simulink model "ALL_JP360_DBW_V6_5_1103"  (R2022a)
settings: Solver=FixedStepAuto  StartTime=0.0  StopTime=inf  FixedStep=0.01  RelTol=1e-3  EnableMultiTasking=on
model workspace (MAT data in the model file):
  g = 9.8
undefined symbols (not defined in the file or in its folder): canChannel, delta_v_p, IPM_Line_C0, IPM_Line_C1, IPM_Line_C2, IPM_Line_C3, M, M_p, MRR_ObjDistX, MRR_ObjDistY, MRR_ObjFusionCamID, MRR_ObjFusionSig, MRR_ObjID, MRR_ObjRelVelX, MRR_ObjRelVelY, MRR_ObjType, MRR_ObjUpdFlg, none, obj_vaild, untracktime, V, videoinput
libraries: canfdmsglib x230, canfdlib x76, slpidlib x24, simulink x18, dspstat3 x14, ctrlSharedLib x1, simulink_extras x1, imaqlib x1, realtime_pacer_lib x1, dspvision x1, visionsinks x1
(part 27 of 55)

== system ALL_JP360_DBW_V6_5_1103/MsgFromCAN/SRR_ADCU_MsgFromCAN/SRR_ADCU_FRR_OBJPos9_0x1AB ==
  SRR_ADCU_FRR_OBJPos9_0x1ABFromInData : Inport  OutDataTypeStr=Bus:CAN_FD_MESSAGE_BUS
  Bus Creator : BusCreator  Inputs=42  OutDataTypeStr=Bus:SRR_ADCU_FRR_OBJPos9_0x1AB  NonVirtualBus=on
  CAN FD Unpack : canfdmsglib/CAN FD Unpack  CANdbFile=V363 SRR Private CAN-V1.3.dbc  MsgList=(none)  MsgName=FRR_OBJPos9_0x1AB  ProtocolMode=CAN FD  MsgIDType=Standard (11-bit identifier)  MsgIdentifier=427  MsgLength=48  SignalInfo={'FRR_CRCCheck_0x1AB','376','16','BE','unsigned','Standard','0','1','0','0','65535';'FRR_OBJ17_Dx','79','13','BE','unsigned','Standard','0','0.0625','-256','-256','255.938';'FRR_OBJ17_Dy','60','11','BE','unsigned','Standard','0','0.125','-128','-128','127.875';'FRR_OBJ17_ExistProb','112','6','BE','unsigned','Standard','0','2','0','0','100';'FRR_OBJ17_HeadingAngle','55','10','BE','unsigned','Standard','0','0.01','-3.14','-3.14','3.14';'FRR_OBJ17_Height','26','9','BE','unsigned','Standard','0','0.01','0','0','5.11';'FRR_OBJ17_Length','33','9','BE','unsigned','Standard','0','0.05','0','0','25.5';'FRR_OBJ17_Measured','126','2','BE','unsigned','Standard','0','1','0','0','3';'FRR_OBJ17_Motion_Status','162','3','BE','unsigned','Standard','0','1','0','0','7';'FRR_OBJ17_ObstacleProb','120','6','BE','unsigned','Standard','0','2','0','0','100';'FRR_OBJ17_RefPointDx','144','13','BE','unsigned','Standard','0','0.0625','-256','-256','255.938';'FRR_OBJ17_RefPointDy','141','11','BE','unsigned','Standard','0','0.125','-128','-128','127.875';'FRR_OBJ17_RefPointLoc','157','3','BE','unsigned','Standard','0','1','0','0','7';'FRR_OBJ17_RelAx','118','9','BE','unsigned','Standard','0','0.0625','-16','-16','15.9375';'FRR_OBJ17_RelAy','111','10','BE','unsigned','Standard','0','0.03125','-16','-16','15.9688';'FRR_OBJ17_RelVx','89','12','BE','unsigned','Standard','0','0.0625','-128','-128','127.938';'FRR_OBJ17_RelVy','85','10','BE','unsigned','Standard','0','0.125','-64','-64','63.875';'FRR_OBJ17_Track_Age','165','8','BE','unsigned','Standard','0','1','0','0','255';'FRR_OBJ17_Track_ID','1','7','BE','unsigned','Standard','0','1','0','0','127';'FRR_OBJ17_Type','14','3','BE','unsigned','Standard','0','1','0','0','7';'FRR_OBJ17_Width','19','11','BE','unsigned','Standard','0','0.01','0','0','12';'FRR_OBJ18_Dx','247','13','BE','unsigned','Standard','0','0.0625','-256','-256','255.938';'FRR_OBJ18_Dy','228','11','BE','unsigned','Standard','0','0.125','-128','-128','127.875';'FRR_OBJ18_ExistProb','280','6','BE','unsigned','Standard','0','2','0','0','100';'FRR_OBJ18_HeadingAngle','223','10','BE','unsigned','Standard','0','0.01','-3.14','-3.14','3.14';'FRR_OBJ18_Height','194','9','BE','unsigned','Standard','0','0.01','0','0','5.11';'FRR_OBJ18_Length','201','9','BE','unsigned','Standard','0','0.05','0','0','25.5';'FRR_OBJ18_Measured','294','2','BE','unsigned','Standard','0','1','0','0','3';'FRR_OBJ18_Motion_Status','330','3','BE','unsigned','Standard','0','1','0','0','7';'FRR_OBJ18_ObstacleProb','288','6','BE','unsigned','Standard','0','2','0','0','100';'FRR_OBJ18_RefPointDx','312','13','BE','unsigned','Standard','0','0.0625','-256','-256','255.938';'FRR_OBJ18_RefPointDy','309','11','BE','unsigned','Standard','0','0.125','-128','-128','127.875';'FRR_OBJ18_RefPointLoc','325','3','BE','unsigned','Standard','0','1','0','0','7';'FRR_OBJ18_RelAx','286','9','BE','unsigned','Standard','0','0.0625','-16','-16','15.9375';'FRR_OBJ18_RelAy','279','10','BE','unsigned','Standard','0','0.03125','-16','-16','15.9688';'FRR_OBJ18_RelVx','257','12','BE','unsigned','Standard','0','0.0625','-128','-128','127.938';'FRR_OBJ18_RelVy','253','10','BE','unsigned','Standard','0','0.125','-64','-64','63.875';'FRR_OBJ18_Track_Age','333','8','BE','unsigned','Standard','0','1','0','0','255';'FRR_OBJ18_Track_ID','169','7','BE','unsigned','Standard','0','1','0','0','127';'FRR_OBJ18_Type','182','3','BE','unsigned','Standard','0','1','0','0','7';'FRR_OBJ18_Width','187','11','BE','unsigned','Standard','0','0.01','0','0','12';'FRR_RollingCounter_0x1AB','360','4','BE','unsigned','Standard','0','1','0','0','15'}  IDPort=off  TimestampPort=off  ErrorPort=off  RemotePort=off  LengthPort=off  StatusPort=off  BRSPort=off  ESIPort=off  DLCPort=off  ApplyMinMax=off
      settings: SourceProductBaseCode=ME,XP,VN  DataFormat=CANdb specified signals
  Data Type Conversion1 : DataTypeConversion  OutDataTypeStr=uint16  SaturateOnIntegerOverflow=off  RndMeth=Floor
  Data Type Conversion{4,8..10,13,19..20,24,28..30,33,39..40,42} (15 alike) : DataTypeConversion  OutDataTypeStr=int8  SaturateOnIntegerOverflow=off  RndMeth=Floor
  Data Type Conversion{2..3,5..7,11..12,14..17,21..23,25..27,31..32,34..37,41} (24 alike) : DataTypeConversion  OutDataTypeStr=single  SaturateOnIntegerOverflow=off  RndMeth=Floor
  Data Type Conversion18 : DataTypeConversion  OutDataTypeStr=uint8  SaturateOnIntegerOverflow=off  RndMeth=Floor
  Data Type Conversion38 : DataTypeConversion  OutDataTypeStr=uint8  SaturateOnIntegerOverflow=off  RndMeth=Floor
  SRR_ADCU_FRR_OBJPos9_0x1ABFromOutData : Outport  OutDataTypeStr=Bus:SRR_ADCU_FRR_OBJPos9_0x1AB
  wires:
  CAN FD Unpack/1 -> Data Type Conversion1/1
  CAN FD Unpack/2 -> Data Type Conversion2/1
  CAN FD Unpack/3 -> Data Type Conversion3/1
  CAN FD Unpack/4 -> Data Type Conversion4/1
  CAN FD Unpack/5 -> Data Type Conversion5/1
  CAN FD Unpack/6 -> Data Type Conversion6/1
  CAN FD Unpack/7 -> Data Type Conversion7/1
  CAN FD Unpack/8 -> Data Type Conversion8/1
  CAN FD Unpack/9 -> Data Type Conversion9/1
  CAN FD Unpack/10 -> Data Type Conversion10/1
  CAN FD Unpack/11 -> Data Type Conversion11/1
  CAN FD Unpack/12 -> Data Type Conversion12/1
  CAN FD Unpack/13 -> Data Type Conversion13/1
  CAN FD Unpack/14 -> Data Type Conversion14/1
  CAN FD Unpack/15 -> Data Type Conversion15/1
  CAN FD Unpack/16 -> Data Type Conversion16/1
  CAN FD Unpack/17 -> Data Type Conversion17/1
  CAN FD Unpack/18 -> Data Type Conversion18/1
  CAN FD Unpack/19 -> Data Type Conversion19/1
  CAN FD Unpack/20 -> Data Type Conversion20/1
  CAN FD Unpack/21 -> Data Type Conversion21/1
  CAN FD Unpack/22 -> Data Type Conversion22/1
  CAN FD Unpack/23 -> Data Type Conversion23/1
  CAN FD Unpack/24 -> Data Type Conversion24/1
  CAN FD Unpack/25 -> Data Type Conversion25/1
  CAN FD Unpack/26 -> Data Type Conversion26/1
  CAN FD Unpack/27 -> Data Type Conversion27/1
  CAN FD Unpack/28 -> Data Type Conversion28/1
  CAN FD Unpack/29 -> Data Type Conversion29/1
  CAN FD Unpack/30 -> Data Type Conversion30/1
  CAN FD Unpack/31 -> Data Type Conversion31/1
  CAN FD Unpack/32 -> Data Type Conversion32/1
  CAN FD Unpack/33 -> Data Type Conversion33/1
  CAN FD Unpack/34 -> Data Type Conversion34/1
  CAN FD Unpack/35 -> Data Type Conversion35/1
  CAN FD Unpack/36 -> Data Type Conversion36/1
  CAN FD Unpack/37 -> Data Type Conversion37/1
  CAN FD Unpack/38 -> Data Type Conversion38/1
  CAN FD Unpack/39 -> Data Type Conversion39/1
  CAN FD Unpack/40 -> Data Type Conversion40/1
  CAN FD Unpack/41 -> Data Type Conversion41/1
  CAN FD Unpack/42 -> Data Type Conversion42/1
  Data Type Conversion1/1 -> Bus Creator/1  "FRR_CRCCheck_0x1AB"
  Data Type Conversion2/1 -> Bus Creator/2  "FRR_OBJ17_Dx"
  Data Type Conversion3/1 -> Bus Creator/3  "FRR_OBJ17_Dy"
  Data Type Conversion4/1 -> Bus Creator/4  "FRR_OBJ17_ExistProb"
  Data Type Conversion5/1 -> Bus Creator/5  "FRR_OBJ17_HeadingAngle"
  Data Type Conversion6/1 -> Bus Creator/6  "FRR_OBJ17_Height"
  Data Type Conversion7/1 -> Bus Creator/7  "FRR_OBJ17_Length"
  Data Type Conversion8/1 -> Bus Creator/8  "FRR_OBJ17_Measured"
  Data Type Conversion9/1 -> Bus Creator/9  "FRR_OBJ17_Motion_Status"
  Data Type Conversion10/1 -> Bus Creator/10  "FRR_OBJ17_ObstacleProb"
  Data Type Conversion11/1 -> Bus Creator/11  "FRR_OBJ17_RefPointDx"
  Data Type Conversion12/1 -> Bus Creator/12  "FRR_OBJ17_RefPointDy"
  Data Type Conversion13/1 -> Bus Creator/13  "FRR_OBJ17_RefPointLoc"
  Data Type Conversion14/1 -> Bus Creator/14  "FRR_OBJ17_RelAx"
  Data Type Conversion15/1 -> Bus Creator/15  "FRR_OBJ17_RelAy"
  Data Type Conversion16/1 -> Bus Creator/16  "FRR_OBJ17_RelVx"
  Data Type Conversion17/1 -> Bus Creator/17  "FRR_OBJ17_RelVy"
  Data Type Conversion18/1 -> Bus Creator/18  "FRR_OBJ17_Track_Age"
  Data Type Conversion19/1 -> Bus Creator/19  "FRR_OBJ17_Track_ID"
  Data Type Conversion20/1 -> Bus Creator/20  "FRR_OBJ17_Type"
  Data Type Conversion21/1 -> Bus Creator/21  "FRR_OBJ17_Width"
  Data Type Conversion22/1 -> Bus Creator/22  "FRR_OBJ18_Dx"
  Data Type Conversion23/1 -> Bus Creator/23  "FRR_OBJ18_Dy"
  Data Type Conversion24/1 -> Bus Creator/24  "FRR_OBJ18_ExistProb"
  Data Type Conversion25/1 -> Bus Creator/25  "FRR_OBJ18_HeadingAngle"
  Data Type Conversion26/1 -> Bus Creator/26  "FRR_OBJ18_Height"
  Data Type Conversion27/1 -> Bus Creator/27  "FRR_OBJ18_Length"
  Data Type Conversion28/1 -> Bus Creator/28  "FRR_OBJ18_Measured"
  Data Type Conversion29/1 -> Bus Creator/29  "FRR_OBJ18_Motion_Status"
  Data Type Conversion30/1 -> Bus Creator/30  "FRR_OBJ18_ObstacleProb"
  Data Type Conversion31/1 -> Bus Creator/31  "FRR_OBJ18_RefPointDx"
  Data Type Conversion32/1 -> Bus Creator/32  "FRR_OBJ18_RefPointDy"
  Data Type Conversion33/1 -> Bus Creator/33  "FRR_OBJ18_RefPointLoc"
  Data Type Conversion34/1 -> Bus Creator/34  "FRR_OBJ18_RelAx"
  Data Type Conversion35/1 -> Bus Creator/35  "FRR_OBJ18_RelAy"
  Data Type Conversion36/1 -> Bus Creator/36  "FRR_OBJ18_RelVx"
  Data Type Conversion37/1 -> Bus Creator/37  "FRR_OBJ18_RelVy"
  Data Type Conversion38/1 -> Bus Creator/38  "FRR_OBJ18_Track_Age"
  Data Type Conversion39/1 -> Bus Creator/39  "FRR_OBJ18_Track_ID"
  Data Type Conversion40/1 -> Bus Creator/40  "FRR_OBJ18_Type"
  Data Type Conversion41/1 -> Bus Creator/41  "FRR_OBJ18_Width"
  Data Type Conversion42/1 -> Bus Creator/42  "FRR_RollingCounter_0x1AB"
  Bus Creator/1 -> SRR_ADCU_FRR_OBJPos9_0x1ABFromOutData/1  "SRR_ADCU_FRR_OBJPos9_0x1ABFromOutData"
  SRR_ADCU_FRR_OBJPos9_0x1ABFromInData/1 -> CAN FD Unpack/1  "SRR_ADCU_FRR_OBJPos9_0x1ABFromInData"

== system ALL_JP360_DBW_V6_5_1103/MsgFromCAN/SRR_ADCU_MsgFromCAN/SRR_ADCU_RLR_AssistSysSt_0x74 ==
  SRR_ADCU_RLR_AssistSysSt_0x74FromInData : Inport  OutDataTypeStr=Bus:CAN_FD_MESSAGE_BUS
  Bus Creator : BusCreator  Inputs=11  OutDataTypeStr=Bus:SRR_ADCU_RLR_AssistSysSt_0x74  NonVirtualBus=on
  CAN FD Unpack : canfdmsglib/CAN FD Unpack  CANdbFile=V363 SRR Private CAN-V1.3.dbc  MsgList=(none)  MsgName=RLR_AssistSysSt_0x74  ProtocolMode=CAN FD  MsgIDType=Standard (11-bit identifier)  MsgIdentifier=116  MsgLength=20  SignalInfo={'RLR_CRCCheck_RLR_AssistSysSt','152','16','BE','unsigned','Standard','0','1','0','0','65535';'RLR_Localtime_Nsec','122','30','BE','unsigned','Standard','0','1','0','0','1073741823';'RLR_Localtime_sec','48','32','BE','unsigned','Standard','0','1','0','0','4294967295';'RLR_RCTBTargetDecel','76','16','BE','unsigned','Standard','0','0.0005','-16','-16','16';'RLR_RCTB_req','60','1','BE','unsigned','Standard','0','1','0','0','1';'RLR_RollingCounter_RLR_AssistSysSt','136','4','BE','unsigned','Standard','0','1','0','0','15';'RLR_SRR_Obj_Failure','5','3','BE','unsigned','Standard','0','1','0','0','7';'RLR_SRR_TiBas','63','1','BE','unsigned','Standard','0','1','0','0','1';'RLR_SRR_TiLeap','62','1','BE','unsigned','Standard','0','1','0','0','1';'RLR_SRR_TiOut','61','1','BE','unsigned','Standard','0','1','0','0','1';'RLR_SRR_alignAngle','8','13','BE','unsigned','Standard','0','0.01','0','0','80'}  IDPort=off  TimestampPort=off  ErrorPort=off  RemotePort=off  LengthPort=off  StatusPort=off  BRSPort=off  ESIPort=off  DLCPort=off  ApplyMinMax=off
      settings: SourceProductBaseCode=ME,XP,VN  DataFormat=CANdb specified signals
  Data Type Conversion1 : DataTypeConversion  OutDataTypeStr=uint16  SaturateOnIntegerOverflow=off  RndMeth=Floor
  Data Type Conversion{5,8..10} (4 alike) : DataTypeConversion  OutDataTypeStr=boolean  SaturateOnIntegerOverflow=off  RndMeth=Floor
  Data Type Conversion11 : DataTypeConversion  OutDataTypeStr=single  SaturateOnIntegerOverflow=off  RndMeth=Floor
  Data Type Conversion2 : DataTypeConversion  OutDataTypeStr=int32  SaturateOnIntegerOverflow=off  RndMeth=Floor
  Data Type Conversion3 : DataTypeConversion  OutDataTypeStr=uint32  SaturateOnIntegerOverflow=off  RndMeth=Floor
  Data Type Conversion4 : DataTypeConversion  OutDataTypeStr=single  SaturateOnIntegerOverflow=off  RndMeth=Floor
  Data Type Conversion6 : DataTypeConversion  OutDataTypeStr=int8  SaturateOnIntegerOverflow=off  RndMeth=Floor
  Data Type Conversion7 : DataTypeConversion  OutDataTypeStr=int8  SaturateOnIntegerOverflow=off  RndMeth=Floor
  SRR_ADCU_RLR_AssistSysSt_0x74FromOutData : Outport  OutDataTypeStr=Bus:SRR_ADCU_RLR_AssistSysSt_0x74
  wires:
  CAN FD Unpack/1 -> Data Type Conversion1/1
  CAN FD Unpack/2 -> Data Type Conversion2/1
  CAN FD Unpack/3 -> Data Type Conversion3/1
  CAN FD Unpack/4 -> Data Type Conversion4/1
  CAN FD Unpack/5 -> Data Type Conversion5/1
  CAN FD Unpack/6 -> Data Type Conversion6/1
  CAN FD Unpack/7 -> Data Type Conversion7/1
  CAN FD Unpack/8 -> Data Type Conversion8/1
  CAN FD Unpack/9 -> Data Type Conversion9/1
  CAN FD Unpack/10 -> Data Type Conversion10/1
  CAN FD Unpack/11 -> Data Type Conversion11/1
  Data Type Conversion1/1 -> Bus Creator/1  "RLR_CRCCheck_RLR_AssistSysSt"
  Data Type Conversion2/1 -> Bus Creator/2  "RLR_Localtime_Nsec"
  Data Type Conversion3/1 -> Bus Creator/3  "RLR_Localtime_sec"
  Data Type Conversion4/1 -> Bus Creator/4  "RLR_RCTBTargetDecel"
  Data Type Conversion5/1 -> Bus Creator/5  "RLR_RCTB_req"
  Data Type Conversion6/1 -> Bus Creator/6  "RLR_RollingCounter_RLR_AssistSysSt"
  Data Type Conversion7/1 -> Bus Creator/7  "RLR_SRR_Obj_Failure"
  Data Type Conversion8/1 -> Bus Creator/8  "RLR_SRR_TiBas"
  Data Type Conversion9/1 -> Bus Creator/9  "RLR_SRR_TiLeap"
  Data Type Conversion10/1 -> Bus Creator/10  "RLR_SRR_TiOut"
  Data Type Conversion11/1 -> Bus Creator/11  "RLR_SRR_alignAngle"
  Bus Creator/1 -> SRR_ADCU_RLR_AssistSysSt_0x74FromOutData/1  "SRR_ADCU_RLR_AssistSysSt_0x74FromOutData"
  SRR_ADCU_RLR_AssistSysSt_0x74FromInData/1 -> CAN FD Unpack/1  "SRR_ADCU_RLR_AssistSysSt_0x74FromInData"

== system ALL_JP360_DBW_V6_5_1103/MsgFromCAN/SRR_ADCU_MsgFromCAN/SRR_ADCU_RLR_Freespace_0x1F1 ==
  SRR_ADCU_RLR_Freespace_0x1F1FromInData : Inport  OutDataTypeStr=Bus:CAN_FD_MESSAGE_BUS
  Bus Creator : BusCreator  Inputs=104  OutDataTypeStr=Bus:SRR_ADCU_RLR_Freespace_0x1F1  NonVirtualBus=on
  CAN FD Unpack : canfdmsglib/CAN FD Unpack  CANdbFile=V363 SRR Private CAN-V1.3.dbc  MsgList=(none)  MsgName=RLR_Freespace_0x1F1  ProtocolMode=CAN FD  MsgIDType=Standard (11-bit identifier)  MsgIdentifier=497  MsgLength=64  SignalInfo={'RLR_CRCCheck_FSP_MSG1','504','16','BE','unsigned','Standard','0','1','0','0','65535';'RLR_FreespaceSectorConfidence1','12','2','BE','unsigned','Standard','0','1','0','0','3';'RLR_FreespaceSectorConfidence10','142','2','BE','unsigned','Standard','0','1','0','0','3';'RLR_FreespaceSectorConfidence11','144','2','BE','unsigned','Standard','0','1','0','0','3';'RLR_FreespaceSectorConfidence12','162','2','BE','unsigned','Standard','0','1','0','0','3';'RLR_FreespaceSectorConfidence13','180','2','BE','unsigned','Standard','0','1','0','0','3';'RLR_FreespaceSectorConfidence14','198','2','BE','unsigned','Standard','0','1','0','0','3';'RLR_FreespaceSectorConfidence15','200','2','BE','unsigned','Standard','0','1','0','0','3';'RLR_FreespaceSectorConfidence16','218','2','BE','unsigned','Standard','0','1','0','0','3';'RLR_FreespaceSectorConfidence17','236','2','BE','unsigned','Standard','0','1','0','0','3';'RLR_FreespaceSectorConfidence18','254','2','BE','unsigned','Standard','0','1','0','0','3';'RLR_FreespaceSectorConfidence19','256','2','BE','unsigned','Standard','0','1','0','0','3';'RLR_FreespaceSectorConfidence2','30','2','BE','unsigned','Standard','0','1','0','0','3';'RLR_FreespaceSectorConfidence20','274','2','BE','unsigned','Standard','0','1','0','0','3';'RLR_FreespaceSectorConfidence21','292','2','BE','unsigned','Standard','0','1','0','0','3';'RLR_FreespaceSectorConfidence22','310','2','BE','unsigned','Standard','0','1','0','0','3';'RLR_FreespaceSectorConfidence23','312','2','BE','unsigned','Standard','0','1','0','0','3';'RLR_FreespaceSectorConfidence24','330','2','BE','unsigned','Standard','0','1','0','0','3';'RLR_FreespaceSectorConfidence25','348','2','BE','unsigned','Standard','0','1','0','0','3';'RLR_FreespaceSectorConfidence26','366','2','BE','unsigned','Standard','0','1','0','0','3';'RLR_FreespaceSectorConfidence27','368','2','BE','unsigned','Standard','0','1','0','0','3';'RLR_FreespaceSectorConfidence28','386','2','BE','unsigned','Standard','0','1','0','0','3';'RLR_FreespaceSectorConfidence29','404','2','BE','unsigned','Standard','0','1','0','0','3';'RLR_FreespaceSectorConfidence3','32','2','BE','unsigned','Standard','0','1','0','0','3';'RLR_FreespaceSectorConfidence30','422','2','BE','unsigned','Standard','0','1','0','0','3';'RLR_FreespaceSectorConfidence31','424','2','BE','unsigned','Standard','0','1','0','0','3';'RLR_FreespaceSectorConfidence32','442','2','BE','unsigned','Standard','0','1','0','0','3';'RLR_FreespaceSectorConfidence33','460','2','BE','unsigned','Standard','0','1','0','0','3';'RLR_FreespaceSectorConfidence34','478','2','BE','unsigned','Standard','0','1','0','0','3';'RLR_FreespaceSectorConfidence4','50','2','BE','unsigned','Standard','0','1','0','0','3';'RLR_FreespaceSectorConfidence5','68','2','BE','unsigned','Standard','0','1','0','0','3';'RLR_FreespaceSectorConfidence6','86','2','BE','unsigned','Standard','0','1','0','0','3';'RLR_FreespaceSectorConfidence7','88','2','BE','unsigned','Standard','0','1','0','0','3';'RLR_FreespaceSectorConfidence8','106','2','BE','unsigned','Standard','0','1','0','0','3';'RLR_FreespaceSectorConfidence9','124','2','BE','unsigned','Standard','0','1','0','0','3';'RLR_FreespaceSectorDistance1','14','10','BE','unsigned','Standard','0','0.1','0','0','100';'RLR_FreespaceSectorDistance10','128','10','BE','unsigned','Standard','0','0.1','0','0','100';'RLR_FreespaceSectorDistance11','146','10','BE','unsigned','Standard','0','0.1','0','0','100';'RLR_FreespaceSectorDistance12','164','10','BE','unsigned','Standard','0','0.1','0','0','100';'RLR_FreespaceSectorDistance13','182','10','BE','unsigned','Standard','0','0.1','0','0','100';'RLR_FreespaceSectorDistance14','184','10','BE','unsigned','Standard','0','0.1','0','0','100';'RLR_FreespaceSectorDistance15','202','10','BE','unsigned','Standard','0','0.1','0','0','100';'RLR_FreespaceSectorDistance16','220','10','BE','unsigned','Standard','0','0.1','0','0','100';'RLR_FreespaceSectorDistance17','238','10','BE','unsigned','Standard','0','0.1','0','0','100';'RLR_FreespaceSectorDistance18','240','10','BE','unsigned','Standard','0','0.1','0','0','100';'RLR_FreespaceSectorDistance19','258','10','BE','unsigned','Standard','0','0.1','0','0','100';'RLR_FreespaceSectorDistance2','16','10','BE','unsigned','Standard','0','0.1','0','0','100';'RLR_FreespaceSectorDistance20','276','10','BE','unsigned','Standard','0','0.1','0','0','100';'RLR_FreespaceSectorDistance21','294','10','BE','unsigned','Standard','0','0.1','0','0','100';'RLR_FreespaceSectorDistance22','296','10','BE','unsigned','Standard','0','0.1','0','0','100';'RLR_FreespaceSectorDistance23','314','10','BE','unsigned','Standard','0','0.1','0','0','100';'RLR_FreespaceSectorDistance24','332','10','BE','unsigned','Standard','0','0.1','0','0','100';'RLR_FreespaceSectorDistance25','350','10','BE','unsigned','Standard','0','0.1','0','0','100';'RLR_FreespaceSectorDistance26','352','10','BE','unsigned','Standard','0','0.1','0','0','100';'RLR_FreespaceSectorDistance27','370','10','BE','unsigned','Standard','0','0.1','0','0','100';'RLR_FreespaceSectorDistance28','388','10','BE','unsigned','Standard','0','0.1','0','0','100';'RLR_FreespaceSectorDistance29','406','10','BE','unsigned','Standard','0','0.1','0','0','100';'RLR_FreespaceSectorDistance3','34','10','BE','unsigned','Standard','0','0.1','0','0','100';'RLR_FreespaceSectorDistance30','408','10','BE','unsigned','Standard','0','0.1','0','0','100';'RLR_FreespaceSectorDistance31','426','10','BE','unsigned','Standard','0','0.1','0','0','100';'RLR_FreespaceSectorDistance32','444','10','BE','unsigned','Standard','0','0.1','0','0','100';'RLR_FreespaceSectorDistance33','462','10','BE','unsigned','Standard','0','0.1','0','0','100';'RLR_FreespaceSectorDistance34','464','10','BE','unsigned','Standard','0','0.1','0','0','100';'RLR_FreespaceSectorDistance4','52','10','BE','unsigned','Standard','0','0.1','0','0','100';'RLR_FreespaceSectorDistance5','70','10','BE','unsigned','Standard','0','0.1','0','0','100';'RLR_FreespaceSectorDistance6','72','10','BE','unsigned','Standard','0','0.1','0','0','100';'RLR_FreespaceSectorDistance7','90','10','BE','unsigned','Standard','0','0.1','0','0','100';'RLR_FreespaceSectorDistance8','108','10','BE','unsigned','Standard','0','0.1','0','0','100';'RLR_FreespaceSectorDistance9','126','10','BE','unsigned','Standard','0','0.1','0','0','100';'RLR_FreespaceSectorKinestate1','10','2','BE','unsigned','Standard','0','1','0','0','3';'RLR_FreespaceSectorKinestate10','140','2','BE','unsigned','Standard','0','1','0','0','3';'RLR_FreespaceSectorKinestate11','158','2','BE','unsigned','Standard','0','1','0','0','3';'RLR_FreespaceSectorKinestate12','160','2','BE','unsigned','Standard','0','1','0','0','3';'RLR_FreespaceSectorKinestate13','178','2','BE','unsigned','Standard','0','1','0','0','3';'RLR_FreespaceSectorKinestate14','196','2','BE','unsigned','Standard','0','1','0','0','3';'RLR_FreespaceSectorKinestate15','214','2','BE','unsigned','Standard','0','1','0','0','3';'RLR_FreespaceSectorKinestate16','216','2','BE','unsigned','Standard','0','1','0','0','3';'RLR_FreespaceSectorKinestate17','234','2','BE','unsigned','Standard','0','1','0','0','3';'RLR_FreespaceSectorKinestate18','252','2','BE','unsigned','Standard','0','1','0','0','3';'RLR_FreespaceSectorKinestate19','270','2','BE','unsigned','Standard','0','1','0','0','3';'RLR_FreespaceSectorKinestate2','28','2','BE','unsigned','Standard','0','1','0','0','3';'RLR_FreespaceSectorKinestate20','272','2','BE','unsigned','Standard','0','1','0','0','3';'RLR_FreespaceSectorKinestate21','290','2','BE','unsigned','Standard','0','1','0','0','3';'RLR_FreespaceSectorKinestate22','308','2','BE','unsigned','Standard','0','1','0','0','3';'RLR_FreespaceSectorKinestate23','326','2','BE','unsigned','Standard','0','1','0','0','3';'RLR_FreespaceSectorKinestate24','328','2','BE','unsigned','Standard','0','1','0','0','3';'RLR_FreespaceSectorKinestate25','346','2','BE','unsigned','Standard','0','1','0','0','3';'RLR_FreespaceSectorKinestate26','364','2','BE','unsigned','Standard','0','1','0','0','3';'RLR_FreespaceSectorKinestate27','382','2','BE','unsigned','Standard','0','1','0','0','3';'RLR_FreespaceSectorKinestate28','384','2','BE','unsigned','Standard','0','1','0','0','3';'RLR_FreespaceSectorKinestate29','402','2','BE','unsigned','Standard','0','1','0','0','3';'RLR_FreespaceSectorKinestate3','46','2','BE','unsigned','Standard','0','1','0','0','3';'RLR_FreespaceSectorKinestate30','420','2','BE','unsigned','Standard','0','1','0','0','3';'RLR_FreespaceSectorKinestate31','438','2','BE','unsigned','Standard','0','1','0','0','3';'RLR_FreespaceSectorKinestate32','440','2','BE','unsigned','Standard','0','1','0','0','3';'RLR_FreespaceSectorKinestate33','458','2','BE','unsigned','Standard','0','1','0','0','3';'RLR_FreespaceSectorKinestate34','476','2','BE','unsigned','Standard','0','1','0','0','3';'RLR_FreespaceSectorKinestate4','48','2','BE','unsigned','Standard','0','1','0','0','3';'RLR_FreespaceSectorKinestate5','66','2','BE','unsigned','Standard','0','1','0','0','3';'RLR_FreespaceSectorKinestate6','84','2','BE','unsigned','Standard','0','1','0','0','3';'RLR_FreespaceSectorKinestate7','102','2','BE','unsigned','Standard','0','1','0','0','3';'RLR_FreespaceSectorKinestate8','104','2','BE','unsigned','Standard','0','1','0','0','3';'RLR_FreespaceSectorKinestate9','122','2','BE','unsigned','Standard','0','1','0','0','3';'RLR_RollingCounter_FSP_MSG1','488','4','BE','unsigned','Standard','0','1','0','0','15'}  IDPort=off  TimestampPort=off  ErrorPort=off  RemotePort=off  LengthPort=off  StatusPort=off  BRSPort=off  ESIPort=off  DLCPort=off  ApplyMinMax=off
      settings: SourceProductBaseCode=ME,XP,VN  DataFormat=CANdb specified signals
  Data Type Conversion1 : DataTypeConversion  OutDataTypeStr=uint16  SaturateOnIntegerOverflow=off  RndMeth=Floor
  Data Type Conversion{2..35,70..104} (69 alike) : DataTypeConversion  OutDataTypeStr=int8  SaturateOnIntegerOverflow=off  RndMeth=Floor
  Data Type Conversion{36..69} (34 alike) : DataTypeConversion  OutDataTypeStr=single  SaturateOnIntegerOverflow=off  RndMeth=Floor
  SRR_ADCU_RLR_Freespace_0x1F1FromOutData : Outport  OutDataTypeStr=Bus:SRR_ADCU_RLR_Freespace_0x1F1
  wires:
  CAN FD Unpack/1 -> Data Type Conversion1/1
  CAN FD Unpack/2 -> Data Type Conversion2/1
  CAN FD Unpack/3 -> Data Type Conversion3/1
  CAN FD Unpack/4 -> Data Type Conversion4/1
  CAN FD Unpack/5 -> Data Type Conversion5/1
  CAN FD Unpack/6 -> Data Type Conversion6/1
  CAN FD Unpack/7 -> Data Type Conversion7/1
  CAN FD Unpack/8 -> Data Type Conversion8/1
  CAN FD Unpack/9 -> Data Type Conversion9/1
  CAN FD Unpack/10 -> Data Type Conversion10/1
  CAN FD Unpack/11 -> Data Type Conversion11/1
  CAN FD Unpack/12 -> Data Type Conversion12/1
  CAN FD Unpack/13 -> Data Type Conversion13/1
  CAN FD Unpack/14 -> Data Type Conversion14/1
  CAN FD Unpack/15 -> Data Type Conversion15/1
  CAN FD Unpack/16 -> Data Type Conversion16/1
  CAN FD Unpack/17 -> Data Type Conversion17/1
  CAN FD Unpack/18 -> Data Type Conversion18/1
  CAN FD Unpack/19 -> Data Type Conversion19/1
  CAN FD Unpack/20 -> Data Type Conversion20/1
  CAN FD Unpack/21 -> Data Type Conversion21/1
  CAN FD Unpack/22 -> Data Type Conversion22/1
  CAN FD Unpack/23 -> Data Type Conversion23/1
  CAN FD Unpack/24 -> Data Type Conversion24/1
  CAN FD Unpack/25 -> Data Type Conversion25/1
  CAN FD Unpack/26 -> Data Type Conversion26/1
  CAN FD Unpack/27 -> Data Type Conversion27/1
  CAN FD Unpack/28 -> Data Type Conversion28/1
  CAN FD Unpack/29 -> Data Type Conversion29/1
  CAN FD Unpack/30 -> Data Type Conversion30/1
  CAN FD Unpack/31 -> Data Type Conversion31/1
  CAN FD Unpack/32 -> Data Type Conversion32/1
  CAN FD Unpack/33 -> Data Type Conversion33/1
  CAN FD Unpack/34 -> Data Type Conversion34/1
  CAN FD Unpack/35 -> Data Type Conversion35/1
  CAN FD Unpack/36 -> Data Type Conversion36/1
  CAN FD Unpack/37 -> Data Type Conversion37/1
  CAN FD Unpack/38 -> Data Type Conversion38/1
  CAN FD Unpack/39 -> Data Type Conversion39/1
  CAN FD Unpack/40 -> Data Type Conversion40/1
  CAN FD Unpack/41 -> Data Type Conversion41/1
  CAN FD Unpack/42 -> Data Type Conversion42/1
  CAN FD Unpack/43 -> Data Type Conversion43/1
  CAN FD Unpack/44 -> Data Type Conversion44/1
  CAN FD Unpack/45 -> Data Type Conversion45/1
  CAN FD Unpack/46 -> Data Type Conversion46/1
  CAN FD Unpack/47 -> Data Type Conversion47/1
  CAN FD Unpack/48 -> Data Type Conversion48/1
  CAN FD Unpack/49 -> Data Type Conversion49/1
  CAN FD Unpack/50 -> Data Type Conversion50/1
  CAN FD Unpack/51 -> Data Type Conversion51/1
  CAN FD Unpack/52 -> Data Type Conversion52/1
  CAN FD Unpack/53 -> Data Type Conversion53/1
  CAN FD Unpack/54 -> Data Type Conversion54/1
  CAN FD Unpack/55 -> Data Type Conversion55/1
  CAN FD Unpack/56 -> Data Type Conversion56/1
  CAN FD Unpack/57 -> Data Type Conversion57/1
  CAN FD Unpack/58 -> Data Type Conversion58/1
  CAN FD Unpack/59 -> Data Type Conversion59/1
  CAN FD Unpack/60 -> Data Type Conversion60/1
  CAN FD Unpack/61 -> Data Type Conversion61/1
  CAN FD Unpack/62 -> Data Type Conversion62/1
  CAN FD Unpack/63 -> Data Type Conversion63/1
  CAN FD Unpack/64 -> Data Type Conversion64/1
  CAN FD Unpack/65 -> Data Type Conversion65/1
  CAN FD Unpack/66 -> Data Type Conversion66/1
  CAN FD Unpack/67 -> Data Type Conversion67/1
  CAN FD Unpack/68 -> Data Type Conversion68/1
  CAN FD Unpack/69 -> Data Type Conversion69/1
  CAN FD Unpack/70 -> Data Type Conversion70/1
  CAN FD Unpack/71 -> Data Type Conversion71/1
  CAN FD Unpack/72 -> Data Type Conversion72/1
  CAN FD Unpack/73 -> Data Type Conversion73/1
  CAN FD Unpack/74 -> Data Type Conversion74/1
  CAN FD Unpack/75 -> Data Type Conversion75/1
  CAN FD Unpack/76 -> Data Type Conversion76/1
  CAN FD Unpack/77 -> Data Type Conversion77/1
  CAN FD Unpack/78 -> Data Type Conversion78/1
  CAN FD Unpack/79 -> Data Type Conversion79/1
  CAN FD Unpack/80 -> Data Type Conversion80/1
  CAN FD Unpack/81 -> Data Type Conversion81/1
  CAN FD Unpack/82 -> Data Type Conversion82/1
  CAN FD Unpack/83 -> Data Type Conversion83/1
  CAN FD Unpack/84 -> Data Type Conversion84/1
  CAN FD Unpack/85 -> Data Type Conversion85/1
  CAN FD Unpack/86 -> Data Type Conversion86/1
  CAN FD Unpack/87 -> Data Type Conversion87/1
  CAN FD Unpack/88 -> Data Type Conversion88/1
  CAN FD Unpack/89 -> Data Type Conversion89/1
  CAN FD Unpack/90 -> Data Type Conversion90/1
  CAN FD Unpack/91 -> Data Type Conversion91/1
  CAN FD Unpack/92 -> Data Type Conversion92/1
  CAN FD Unpack/93 -> Data Type Conversion93/1
  CAN FD Unpack/94 -> Data Type Conversion94/1
  CAN FD Unpack/95 -> Data Type Conversion95/1
  CAN FD Unpack/96 -> Data Type Conversion96/1
  CAN FD Unpack/97 -> Data Type Conversion97/1
  CAN FD Unpack/98 -> Data Type Conversion98/1
  CAN FD Unpack/99 -> Data Type Conversion99/1
  CAN FD Unpack/100 -> Data Type Conversion100/1
  CAN FD Unpack/101 -> Data Type Conversion101/1
  CAN FD Unpack/102 -> Data Type Conversion102/1
  CAN FD Unpack/103 -> Data Type Conversion103/1
  CAN FD Unpack/104 -> Data Type Conversion104/1
  Data Type Conversion1/1 -> Bus Creator/1  "RLR_CRCCheck_FSP_MSG1"
  Data Type Conversion2/1 -> Bus Creator/2  "RLR_FreespaceSectorConfidence1"
  Data Type Conversion3/1 -> Bus Creator/3  "RLR_FreespaceSectorConfidence10"
  Data Type Conversion4/1 -> Bus Creator/4  "RLR_FreespaceSectorConfidence11"
  Data Type Conversion5/1 -> Bus Creator/5  "RLR_FreespaceSectorConfidence12"
  Data Type Conversion6/1 -> Bus Creator/6  "RLR_FreespaceSectorConfidence13"
  Data Type Conversion7/1 -> Bus Creator/7  "RLR_FreespaceSectorConfidence14"
  Data Type Conversion8/1 -> Bus Creator/8  "RLR_FreespaceSectorConfidence15"
  Data Type Conversion9/1 -> Bus Creator/9  "RLR_FreespaceSectorConfidence16"
  Data Type Conversion10/1 -> Bus Creator/10  "RLR_FreespaceSectorConfidence17"
  Data Type Conversion11/1 -> Bus Creator/11  "RLR_FreespaceSectorConfidence18"
  Data Type Conversion12/1 -> Bus Creator/12  "RLR_FreespaceSectorConfidence19"
  Data Type Conversion13/1 -> Bus Creator/13  "RLR_FreespaceSectorConfidence2"
  Data Type Conversion14/1 -> Bus Creator/14  "RLR_FreespaceSectorConfidence20"
  Data Type Conversion15/1 -> Bus Creator/15  "RLR_FreespaceSectorConfidence21"
  Data Type Conversion16/1 -> Bus Creator/16  "RLR_FreespaceSectorConfidence22"
  Data Type Conversion17/1 -> Bus Creator/17  "RLR_FreespaceSectorConfidence23"
  Data Type Conversion18/1 -> Bus Creator/18  "RLR_FreespaceSectorConfidence24"
  Data Type Conversion19/1 -> Bus Creator/19  "RLR_FreespaceSectorConfidence25"
  Data Type Conversion20/1 -> Bus Creator/20  "RLR_FreespaceSectorConfidence26"
  Data Type Conversion21/1 -> Bus Creator/21  "RLR_FreespaceSectorConfidence27"
  Data Type Conversion22/1 -> Bus Creator/22  "RLR_FreespaceSectorConfidence28"
  Data Type Conversion23/1 -> Bus Creator/23  "RLR_FreespaceSectorConfidence29"
  Data Type Conversion24/1 -> Bus Creator/24  "RLR_FreespaceSectorConfidence3"
  Data Type Conversion25/1 -> Bus Creator/25  "RLR_FreespaceSectorConfidence30"
  Data Type Conversion26/1 -> Bus Creator/26  "RLR_FreespaceSectorConfidence31"
  Data Type Conversion27/1 -> Bus Creator/27  "RLR_FreespaceSectorConfidence32"
  Data Type Conversion28/1 -> Bus Creator/28  "RLR_FreespaceSectorConfidence33"
  Data Type Conversion29/1 -> Bus Creator/29  "RLR_FreespaceSectorConfidence34"
  Data Type Conversion30/1 -> Bus Creator/30  "RLR_FreespaceSectorConfidence4"
  Data Type Conversion31/1 -> Bus Creator/31  "RLR_FreespaceSectorConfidence5"
  Data Type Conversion32/1 -> Bus Creator/32  "RLR_FreespaceSectorConfidence6"
  Data Type Conversion33/1 -> Bus Creator/33  "RLR_FreespaceSectorConfidence7"
  Data Type Conversion34/1 -> Bus Creator/34  "RLR_FreespaceSectorConfidence8"
  Data Type Conversion35/1 -> Bus Creator/35  "RLR_FreespaceSectorConfidence9"
  Data Type Conversion36/1 -> Bus Creator/36  "RLR_FreespaceSectorDistance1"
  Data Type Conversion37/1 -> Bus Creator/37  "RLR_FreespaceSectorDistance10"
  Data Type Conversion38/1 -> Bus Creator/38  "RLR_FreespaceSectorDistance11"
  Data Type Conversion39/1 -> Bus Creator/39  "RLR_FreespaceSectorDistance12"
  Data Type Conversion40/1 -> Bus Creator/40  "RLR_FreespaceSectorDistance13"
  Data Type Conversion41/1 -> Bus Creator/41  "RLR_FreespaceSectorDistance14"
  Data Type Conversion42/1 -> Bus Creator/42  "RLR_FreespaceSectorDistance15"
  Data Type Conversion43/1 -> Bus Creator/43  "RLR_FreespaceSectorDistance16"
  Data Type Conversion44/1 -> Bus Creator/44  "RLR_FreespaceSectorDistance17"
  Data Type Conversion45/1 -> Bus Creator/45  "RLR_FreespaceSectorDistance18"
  Data Type Conversion46/1 -> Bus Creator/46  "RLR_FreespaceSectorDistance19"
  Data Type Conversion47/1 -> Bus Creator/47  "RLR_FreespaceSectorDistance2"
  Data Type Conversion48/1 -> Bus Creator/48  "RLR_FreespaceSectorDistance20"
  Data Type Conversion49/1 -> Bus Creator/49  "RLR_FreespaceSectorDistance21"
  Data Type Conversion50/1 -> Bus Creator/50  "RLR_FreespaceSectorDistance22"
  Data Type Conversion51/1 -> Bus Creator/51  "RLR_FreespaceSectorDistance23"
  Data Type Conversion52/1 -> Bus Creator/52  "RLR_FreespaceSectorDistance24"
  Data Type Conversion53/1 -> Bus Creator/53  "RLR_FreespaceSectorDistance25"
  Data Type Conversion54/1 -> Bus Creator/54  "RLR_FreespaceSectorDistance26"
  Data Type Conversion55/1 -> Bus Creator/55  "RLR_FreespaceSectorDistance27"
  Data Type Conversion56/1 -> Bus Creator/56  "RLR_FreespaceSectorDistance28"
  Data Type Conversion57/1 -> Bus Creator/57  "RLR_FreespaceSectorDistance29"
  Data Type Conversion58/1 -> Bus Creator/58  "RLR_FreespaceSectorDistance3"
  Data Type Conversion59/1 -> Bus Creator/59  "RLR_FreespaceSectorDistance30"
  Data Type Conversion60/1 -> Bus Creator/60  "RLR_FreespaceSectorDistance31"
  Data Type Conversion61/1 -> Bus Creator/61  "RLR_FreespaceSectorDistance32"
  Data Type Conversion62/1 -> Bus Creator/62  "RLR_FreespaceSectorDistance33"
  Data Type Conversion63/1 -> Bus Creator/63  "RLR_FreespaceSectorDistance34"
  Data Type Conversion64/1 -> Bus Creator/64  "RLR_FreespaceSectorDistance4"
  Data Type Conversion65/1 -> Bus Creator/65  "RLR_FreespaceSectorDistance5"
  Data Type Conversion66/1 -> Bus Creator/66  "RLR_FreespaceSectorDistance6"
  Data Type Conversion67/1 -> Bus Creator/67  "RLR_FreespaceSectorDistance7"
  Data Type Conversion68/1 -> Bus Creator/68  "RLR_FreespaceSectorDistance8"
  Data Type Conversion69/1 -> Bus Creator/69  "RLR_FreespaceSectorDistance9"
  Data Type Conversion70/1 -> Bus Creator/70  "RLR_FreespaceSectorKinestate1"
  Data Type Conversion71/1 -> Bus Creator/71  "RLR_FreespaceSectorKinestate10"
  Data Type Conversion72/1 -> Bus Creator/72  "RLR_FreespaceSectorKinestate11"
  Data Type Conversion73/1 -> Bus Creator/73  "RLR_FreespaceSectorKinestate12"
  Data Type Conversion74/1 -> Bus Creator/74  "RLR_FreespaceSectorKinestate13"
  Data Type Conversion75/1 -> Bus Creator/75  "RLR_FreespaceSectorKinestate14"
  Data Type Conversion76/1 -> Bus Creator/76  "RLR_FreespaceSectorKinestate15"
  Data Type Conversion77/1 -> Bus Creator/77  "RLR_FreespaceSectorKinestate16"
  Data Type Conversion78/1 -> Bus Creator/78  "RLR_FreespaceSectorKinestate17"
  Data Type Conversion79/1 -> Bus Creator/79  "RLR_FreespaceSectorKinestate18"
  Data Type Conversion80/1 -> Bus Creator/80  "RLR_FreespaceSectorKinestate19"
  Data Type Conversion81/1 -> Bus Creator/81  "RLR_FreespaceSectorKinestate2"
  Data Type Conversion82/1 -> Bus Creator/82  "RLR_FreespaceSectorKinestate20"
  Data Type Conversion83/1 -> Bus Creator/83  "RLR_FreespaceSectorKinestate21"
  Data Type Conversion84/1 -> Bus Creator/84  "RLR_FreespaceSectorKinestate22"
  Data Type Conversion85/1 -> Bus Creator/85  "RLR_FreespaceSectorKinestate23"
  Data Type Conversion86/1 -> Bus Creator/86  "RLR_FreespaceSectorKinestate24"
  Data Type Conversion87/1 -> Bus Creator/87  "RLR_FreespaceSectorKinestate25"
  Data Type Conversion88/1 -> Bus Creator/88  "RLR_FreespaceSectorKinestate26"
  Data Type Conversion89/1 -> Bus Creator/89  "RLR_FreespaceSectorKinestate27"
  Data Type Conversion90/1 -> Bus Creator/90  "RLR_FreespaceSectorKinestate28"
  Data Type Conversion91/1 -> Bus Creator/91  "RLR_FreespaceSectorKinestate29"
  Data Type Conversion92/1 -> Bus Creator/92  "RLR_FreespaceSectorKinestate3"
  Data Type Conversion93/1 -> Bus Creator/93  "RLR_FreespaceSectorKinestate30"
  Data Type Conversion94/1 -> Bus Creator/94  "RLR_FreespaceSectorKinestate31"
  Data Type Conversion95/1 -> Bus Creator/95  "RLR_FreespaceSectorKinestate32"
  Data Type Conversion96/1 -> Bus Creator/96  "RLR_FreespaceSectorKinestate33"
  Data Type Conversion97/1 -> Bus Creator/97  "RLR_FreespaceSectorKinestate34"
  Data Type Conversion98/1 -> Bus Creator/98  "RLR_FreespaceSectorKinestate4"
  Data Type Conversion99/1 -> Bus Creator/99  "RLR_FreespaceSectorKinestate5"
  Data Type Conversion100/1 -> Bus Creator/100  "RLR_FreespaceSectorKinestate6"
  Data Type Conversion101/1 -> Bus Creator/101  "RLR_FreespaceSectorKinestate7"
  Data Type Conversion102/1 -> Bus Creator/102  "RLR_FreespaceSectorKinestate8"
  Data Type Conversion103/1 -> Bus Creator/103  "RLR_FreespaceSectorKinestate9"
  Data Type Conversion104/1 -> Bus Creator/104  "RLR_RollingCounter_FSP_MSG1"
  Bus Creator/1 -> SRR_ADCU_RLR_Freespace_0x1F1FromOutData/1  "SRR_ADCU_RLR_Freespace_0x1F1FromOutData"
  SRR_ADCU_RLR_Freespace_0x1F1FromInData/1 -> CAN FD Unpack/1  "SRR_ADCU_RLR_Freespace_0x1F1FromInData"
